simulink model "L4A3_simu"  (R2021b)
settings: Solver=VariableStepAuto  StartTime=0.0  StopTime=60  MaxStep=0.0001  RelTol=1e-3
values from neighbouring files (symbols this model uses):
  C_2 = 97e-9    (= 9.7e-08)    [L4A3.m]
  C_3 = 5.8e-9    (= 5.8e-09)    [L4A3.m]
  R_2 = 10e3    (= 10000)    [L4A3.m]
  R_3 = 10e3    (= 10000)    [L4A3.m]
  R_4 = 1e3    (= 1000)    [L4A3.m]
  R_5 = 10e3    (= 10000)    [L4A3.m]
  R_6 = 2200    [L4A3.m]
settings Model: Creator=tobia  LastModifiedBy=tobia

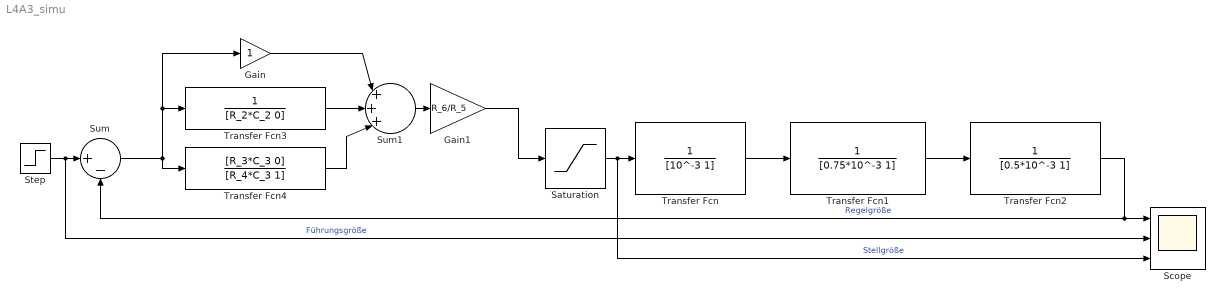
== system L4A3_simu ==
  Gain : Gain
  Gain1 : Gain  Gain=R_6/R_5
  Saturation : Saturate  UpperLimit=12  LowerLimit=-12
  Scope : Scope  NumInputPorts=3
  Step : Step  Time=0  After=5  SampleTime=0
  Sum : Sum  Inputs=|+-
  Sum1 : Sum  Inputs=|+++|
  Transfer Fcn : TransferFcn  Denominator=[10^-3 1]
  Transfer Fcn1 : TransferFcn  Denominator=[0.75*10^-3 1]
  Transfer Fcn2 : TransferFcn  Denominator=[0.5*10^-3 1]
  Transfer Fcn3 : TransferFcn  Denominator=[R_2*C_2 0]
  Transfer Fcn4 : TransferFcn  Numerator=[R_3*C_3 0]  Denominator=[R_4*C_3 1]
  wires:
  Transfer Fcn/1 -> Transfer Fcn1/1
  Transfer Fcn1/1 -> Transfer Fcn2/1
  Saturation/1 -> Scope/3, Transfer Fcn/1  "Stellgröße"
  Transfer Fcn2/1 -> Sum/2, Scope/1  "Regelgröße"
  Step/1 -> Scope/2, Sum/1  "Führungsgröße"
  Sum/1 -> Gain/1, Transfer Fcn3/1, Transfer Fcn4/1
  Transfer Fcn3/1 -> Sum1/2
  Gain/1 -> Sum1/1
  Transfer Fcn4/1 -> Sum1/3
  Sum1/1 -> Gain1/1
  Gain1/1 -> Saturation/1
